simulink library "CTRL_LO_ST2"  (R2023b)
settings: Solver=VariableStepAuto  StartTime=0.0  StopTime=10.0  RelTol=1e-3
undefined symbols (not defined in the file or in its folder): CTRL_LO_p_TqMotLoLim_Nm, CTRL_LO_p_TqMotUpLim_Nm, CTRL_LO_ST2_p_SwtTqFrReRat_na, CTRL_LO_ST2_p_SwtTqLeRiRat_na, CTRL_LO_ST2_p_TqFrReRat1_na, CTRL_LO_ST2_p_TqFrReRat2_na, CTRL_LO_ST2_p_TqFrReRat3_na, CTRL_LO_ST2_p_TqLeRiRat1_na, CTRL_LO_ST2_p_TqLeRiRat2_na, CTRL_LO_ST2_p_TqLeRiRat3_na, CTRL_LO_ST2_p_TqLeRiRat4_na
libraries: simulink x1
settings Model: Creator=blatak  LastModifiedBy=blatak

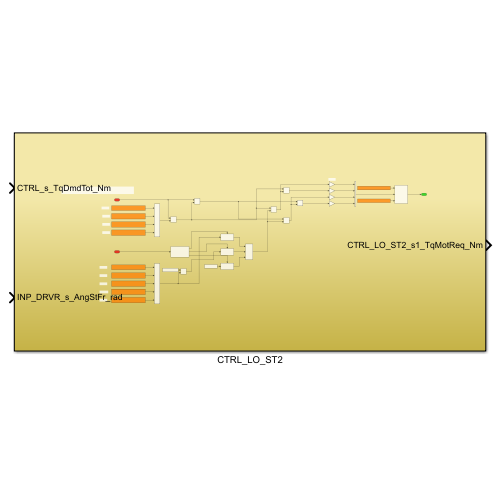
[thumbnail: Simulink's stored preview of the top-level diagram]
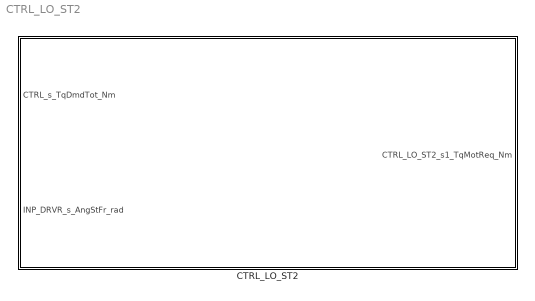
== system CTRL_LO_ST2 ==
  CTRL_LO_ST2 : Subsystem

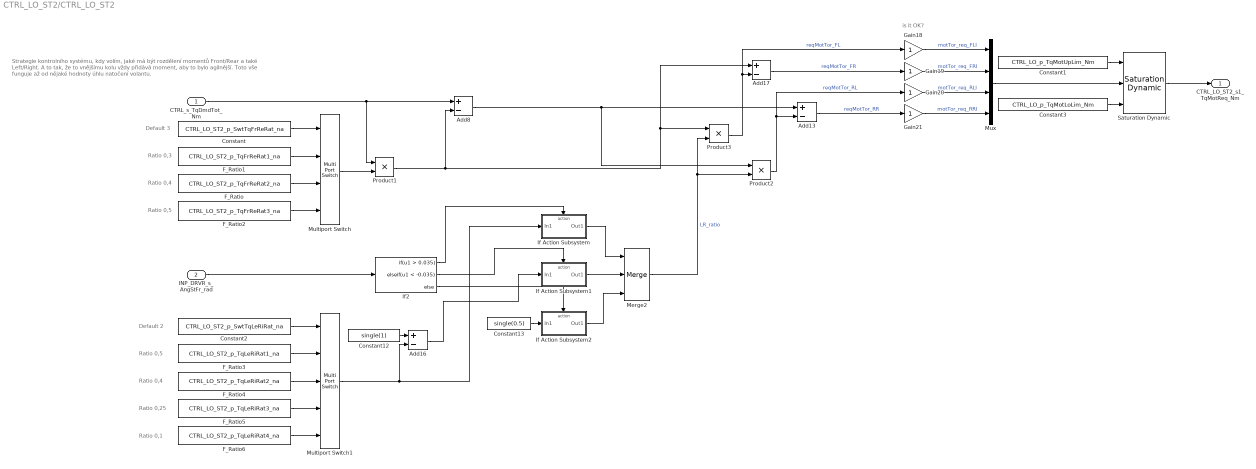
== system CTRL_LO_ST2/CTRL_LO_ST2 ==
  note: Strategie kontrolního systému, kdy volím, jaké má být rozdělení momentů Front/Rear
      | a také Left/Right. A to tak, že to vnějšímu kolu vždy přidává moment, aby to bylo agilnější.
      | Toto vše funguje až od nějaké hodnoty úhlu natočení volantu.
  note: is it OK?
  note: Default 3
  note: Ratio 0,3
  note: Ratio 0,4
  note: Ratio 0,5
  note: Default 2
  note: Ratio 0,5
  note: Ratio 0,4
  note: Ratio 0,25
  note: Ratio 0,1
  CTRL_s_TqDmdTot_Nm : Inport
  INP_DRVR_s_AngStFr_rad : Inport  Port=2
  Add{8,13,16..17} (4 alike) : Sum  Inputs=+-
  Constant : Constant  Value=CTRL_LO_ST2_p_SwtTqFrReRat_na
  Constant1 : Constant  Value=CTRL_LO_p_TqMotUpLim_Nm
  Constant12 : Constant  Value=single(1)
  Constant13 : Constant  Value=single(0.5)
  Constant2 : Constant  Value=CTRL_LO_ST2_p_SwtTqLeRiRat_na
  Constant3 : Constant  Value=CTRL_LO_p_TqMotLoLim_Nm
  F_Ratio : Constant  Value=CTRL_LO_ST2_p_TqFrReRat2_na
  F_Ratio1 : Constant  Value=CTRL_LO_ST2_p_TqFrReRat1_na
  F_Ratio2 : Constant  Value=CTRL_LO_ST2_p_TqFrReRat3_na
  F_Ratio3 : Constant  Value=CTRL_LO_ST2_p_TqLeRiRat1_na
  F_Ratio4 : Constant  Value=CTRL_LO_ST2_p_TqLeRiRat2_na
  F_Ratio5 : Constant  Value=CTRL_LO_ST2_p_TqLeRiRat3_na
  F_Ratio6 : Constant  Value=CTRL_LO_ST2_p_TqLeRiRat4_na
  Gain{18..21} (4 alike) : Gain
  If Action Subsystem : Subsystem  TreatAsAtomicUnit=on
  If Action Subsystem1 : Subsystem  TreatAsAtomicUnit=on
  If Action Subsystem2 : Subsystem  TreatAsAtomicUnit=on
  If2 : If  IfExpression=u1 > 0.035  ElseIfExpressions=u1 < -0.035
  Merge2 : Merge  Inputs=3
  Multiport Switch : MultiPortSwitch  SaturateOnIntegerOverflow=off  InputSameDT=off
  Multiport Switch1 : MultiPortSwitch  Inputs=4  SaturateOnIntegerOverflow=off  InputSameDT=off
  Mux : Mux
  Product1 : Product
  Product2 : Product
  Product3 : Product
  Saturation Dynamic : simulink/Discontinuities/Saturation Dynamic  OutMin=[]  OutMax=[]  OutDataTypeStr=Inherit: Same as second input  OutDataType=fixdt(1, 16)  OutScaling=2^-10  DoSatur=off
  CTRL_LO_ST2_s1_TqMotReq_Nm : Outport
  wires:
  Product3/1 -> Gain18/1, Add17/2  "reqMotTor_FL"
  Add8/1 -> Product2/1, Add13/1
  If Action Subsystem2/1(Out1) -> Merge2/3
  Gain21/1 -> Mux/4  "motTor_req_RRI"
  Constant/1 -> Multiport Switch/1
  If2/3 -> If Action Subsystem2/Action
  Gain19/1 -> Mux/2  "motTor_req_FRI"
  Product1/1 -> Add8/2, Product3/1, Add17/1
  If Action Subsystem/1(Out1) -> Merge2/1
  Constant13/1 -> If Action Subsystem2/1(In1)
  F_Ratio1/1 -> Multiport Switch/2
  Constant12/1 -> Add16/1
  INP_DRVR_s_AngStFr_rad/1 -> If2/1
  Product2/1 -> Add13/2, Gain20/1  "reqMotTor_RL"
  F_Ratio2/1 -> Multiport Switch/4
  If2/2 -> If Action Subsystem1/Action
  If2/1 -> If Action Subsystem/Action
  Add13/1 -> Gain21/1  "reqMotTor_RR"
  F_Ratio4/1 -> Multiport Switch1/3
  Gain18/1 -> Mux/1  "motTor_req_FLI"
  Constant2/1 -> Multiport Switch1/1
  CTRL_s_TqDmdTot_Nm/1 -> Product1/1, Add8/1
  Gain20/1 -> Mux/3  "motTor_req_RLI"
  F_Ratio3/1 -> Multiport Switch1/2
  F_Ratio/1 -> Multiport Switch/3
  Multiport Switch1/1 -> If Action Subsystem/1(In1), Add16/2
  Merge2/1 -> Product3/2, Product2/2  "LR_ratio"
  Add17/1 -> Gain19/1  "reqMotTor_FR"
  F_Ratio6/1 -> Multiport Switch1/5
  F_Ratio5/1 -> Multiport Switch1/4
  Multiport Switch/1 -> Product1/2
  Add16/1 -> If Action Subsystem1/1(In1)
  If Action Subsystem1/1(Out1) -> Merge2/2
  Constant1/1 -> Saturation Dynamic/1
  Constant3/1 -> Saturation Dynamic/3
  Mux/1 -> Saturation Dynamic/2
  Saturation Dynamic/1 -> CTRL_LO_ST2_s1_TqMotReq_Nm/1

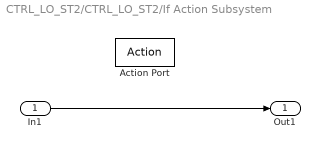
== system CTRL_LO_ST2/CTRL_LO_ST2/If Action Subsystem ==
  In1 : Inport
  Action Port : ActionPort  ActionPortLabel=if(u1 > 0.035)
  Out1 : Outport
  wires:
  In1/1 -> Out1/1

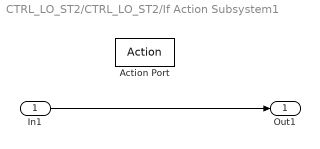
== system CTRL_LO_ST2/CTRL_LO_ST2/If Action Subsystem1 ==
  In1 : Inport
  Action Port : ActionPort  ActionPortLabel=elseif(u1 < -0.035)
  Out1 : Outport
  wires:
  In1/1 -> Out1/1

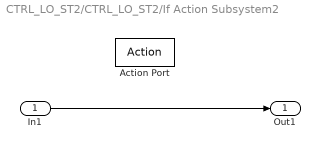
== system CTRL_LO_ST2/CTRL_LO_ST2/If Action Subsystem2 ==
  In1 : Inport
  Action Port : ActionPort  ActionPortLabel=else
  Out1 : Outport
  wires:
  In1/1 -> Out1/1
